simulink model "example_temperature_regulation"  (R2021a)
settings: Solver=ode15s  StartTime=0.0  StopTime=10.0  FixedStep=0.1  RelTol=1e-3  EnableMultiTasking=on
settings Model: Creator=acalame  LastModifiedBy=gabin
settings SolverCC: AlgebraicLoopSolver=TrustRegion  AutoInsertRateTranBlk=on
settings DataIOCC: LimitDataPoints=on
settings OptimizationCC: LifeSpan=inf
settings DebuggingCC: AllowSymbolicDim=off  SFUnexpectedBacktrackingDiag=warning  SFNoUnconditionalDefaultTransitionDiag=warning  SFExecutionAtInitializationDiag=none  ArithmeticOperatorsInVariantConditions=warning
settings SFSimCC: SimUseLocalCustomCode=off  CustomCodeUndefinedFunction=UseInterfaceOnly
settings RTWCC: RTWUseLocalCustomCode=off
settings CodeAppCC: StateflowObjectComments=on
settings GRTTargetCC: TargetLangStandard=C89/C90 (ANSI)
settings ConfigComp: CovMetricSettings=dw  CovSaveCumulativeToWorkspaceVar=on  CovSaveSingleToWorkspaceVar=on  CovExternalEMLEnable=off  CovSFcnEnable=off

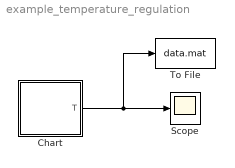
== system example_temperature_regulation ==
  Chart : Stateflow chart  TreatAsAtomicUnit=on
  Scope : Scope
  To File : ToFile  Filename=data.mat  MatrixName=X  SaveFormat=Timeseries
  wires:
  Chart/1(T) -> Scope/1, To File/1

== stateflow chart example_temperature_regulation/Chart ==
  settings: updateMethod=CONTINUOUS
  state chauf
    during:
    T_dot = 10 - 0.4*T;
  state arret
    during:
    T_dot = 0 - 0.45*T;
  (default) -> chauf : {T=10}
  chauf -> arret : [T>=21]
  arret -> chauf : [T<=19]
  data: T output =10
  data T settings: updateMethod=SF_CONTINUOUS_TIME_DATA
